simulink model "BuckConvAveMod"  (R2022a)
settings: Solver=VariableStepAuto  StartTime=0.0  StopTime=10  RelTol=1e-3
values from neighbouring files (symbols this model uses):
  C = 10e-5    (= 0.0001)    [Premodeling.m]
  L = 100.8e-3    (= 0.1008)    [Premodeling.m]
  R = 100    [Premodeling.m]
  Vin = 24    [Premodeling.m]
libraries: spsBuckConverterLib x1, spsCurrentMeasurementLib x1, spsDCVoltageSourceLib x1, spsGroundLib x1, spsParallelRLCBranchLib x1, spsSeriesRLCBranchLib x1, spsVoltageMeasurementLib x1, spspowerguiLib x1
settings Model: Creator=Andrew  LastModifiedBy=Andrew

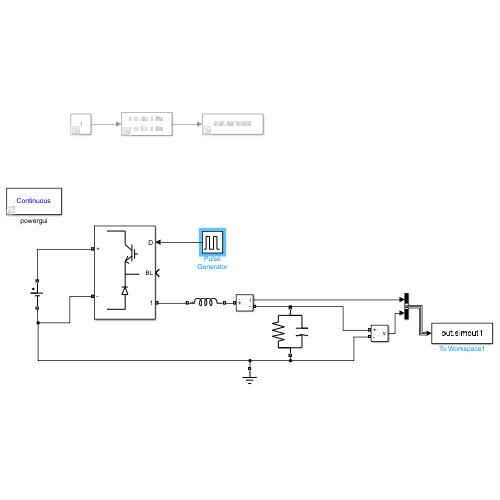
[thumbnail: Simulink's stored preview of the top-level diagram]
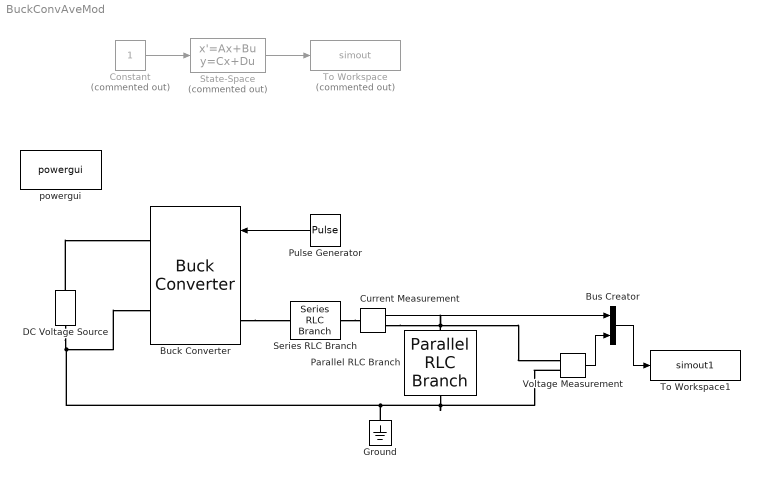
== system BuckConvAveMod ==
  Buck Converter : spsBuckConverterLib/Buck Converter  ModelType=Average model (D-controlled)  Ron=1e-3  Rs=1e6  Cs=inf  Vforward=[0,0]  Ron_Diode=1e-3  Rs_Diode=1e6  Cs_Diode=inf  Vf_Diode=1e-3  Rs_CurrentSource=inf  Ron_ACsource=1e-3
      settings: SourceProductBaseCode=PS
  Bus Creator : BusCreator  Inputs=2
  Constant : Constant  Commented=on
  Current Measurement : spsCurrentMeasurementLib/Current Measurement  PhasorSimulation=off  OutputType=Complex  PSBequivalent=0
  DC Voltage Source : spsDCVoltageSourceLib/DC Voltage Source  Amplitude=Vin  Measurements=None
  Ground : spsGroundLib/Ground  LConnTagsString=a
  Parallel RLC Branch : spsParallelRLCBranchLib/Parallel RLC Branch  LConnTagsString=a  RConnTagsString=__new0  BranchType=RC  Resistance=R  Inductance=0  SetiL0=off  InitialCurrent=0  Capacitance=C  Setx0=off  InitialVoltage=0  Measurements=None
  Pulse Generator : DiscretePulseGenerator  PulseType=Time based  Period=0.001  PulseWidth=50
  Series RLC Branch : spsSeriesRLCBranchLib/Series RLC Branch  LConnTagsString=__new0  RConnTagsString=__new0  BranchType=L  Resistance=1  Inductance=L  SetiL0=off  InitialCurrent=0  Capacitance=1e-6  Setx0=off  InitialVoltage=0  Measurements=None
  State-Space : StateSpace  Commented=on  A=[0 -1/L; 1/C -1/(R*C)]  B=[Vin/L; 0]  C=[0 1]  D=0  InitialCondition=0
  To Workspace : ToWorkspace  Commented=on  VariableName=simout  SaveFormat=Timeseries  SampleTime=-1
  To Workspace1 : ToWorkspace  VariableName=simout1  SaveFormat=Timeseries  SampleTime=-1
  Voltage Measurement : spsVoltageMeasurementLib/Voltage Measurement  PhasorSimulation=off  OutputType=Complex  PSBequivalent=0
  powergui : spspowerguiLib/powergui  Priority=1  SimulationMode=Continuous  SampleTime=50e-6  frequency=60  Iterations=50  frequencyindice=0  Pbase=100e6  ErrMax=1e-4  UnitsV=kV  UnitsW=MW  buscounter=0  FunctionMessages=off  echomessages=off  EnableUseOfTLC=off  CurrentSourceSwitches=off  DisableSnubberDevices=off  DisableRonSwitches=off  DisableVfSwitches=off  DisplayEquations=off  AutomaticDiscreteSolvers=off  SolverType=Tustin/Backward Euler (TBE)  Interpol=off  ExternalGateDelay=off  methode=off  Ts=100  x0status=blocks  SPID=on  SwTol=0  HookPort=off  NonlinearTolerance=1e-4  nMaxIteration=100  ContinueOnMaxIteration=off  RestoreLinks=warning  ResistiveCurrentMeasurement=off  Frange=[0:2:500]  Ylog=off  Xlog=on  ShowGrid=off  save=off  variable=ZData  structure=0  ZoomFFT=off  StartTime=0.0  cycles=1  DisplayStyle=1  fundamental=60  FreqAxis=off  MaxFrequency=1000  frequencyindicesteady=1  RmsSteady=1  display=off
  wires:
  Constant/1 -> State-Space/1
  State-Space/1 -> To Workspace/1
  Voltage Measurement/1 -> Bus Creator/2
  Current Measurement/1 -> Bus Creator/1
  Bus Creator/1 -> To Workspace1/1
  Pulse Generator/1 -> Buck Converter/1
  connections:
  DC Voltage Source/RConn1 -- Buck Converter/RConn1
  DC Voltage Source/LConn1 -- Parallel RLC Branch/RConn1 -- Voltage Measurement/LConn2 -- Ground/LConn1 -- Buck Converter/RConn2
  Buck Converter/LConn1 -- Series RLC Branch/LConn1
  Series RLC Branch/RConn1 -- Current Measurement/LConn1
  Current Measurement/RConn1 -- Parallel RLC Branch/LConn1 -- Voltage Measurement/LConn1
